simulink model "Controller_PP"  (R2021a)
settings: Solver=FixedStepDiscrete  StartTime=0.0  StopTime=inf  FixedStep=0.05  RelTol=1e-3
PostLoadFcn:
  | , if any(exist('dsrtsu_mdlpostloadfcn', 'file') == [2, 3, 6]), try dsrtsu_mdlpostloadfcn('Execute', bdroot); catch fprintf('Error in PostLoadFcn (dsrtsu_mdlpostloadfcn) for model "%s":\n %s\n', bdroot, lasterr); end, end,
model workspace (MAT data in the model file):
  DLC_kr = [-5.84862481044e-05 -6.43095507895e-05 -7.01328534794e-05 -7.5956156174e-05 -8.17794588731e-05 -8.76027615758e-05 -9.34260642811e-05 -9.92493669872e-05 -0.000105072669692 -0.000110895972393 -0.000116719275087 -0.000122542545808 ... (2080 elements, 1x2080)]
  DLC_thetar = [1.57172954906 1.57172588114 1.57172186534 1.57171750165 1.57171279008 1.57170773062 1.57170232328 1.57169656806 1.57169046495 1.57168401395 1.57167721507 1.57167006831 ... (2080 elements, 1x2080)]
  DLC_xr = [-0.00056695162723 -0.000622594591628 -0.000678008043004 -0.000733171198692 -0.000788063276025 -0.000842663492338 -0.000896951064963 -0.000950905211235 -0.00100450514849 -0.00105773009405 -0.00111055926527 -0.00116297187948 ... (2080 elements, 1x2080)]
  DLC_yr = [0.59999973213 0.659739817002 0.719479902091 0.779219987412 0.838960072984 0.898700158824 0.958440244948 1.01818033138 1.07792041812 1.1376605052 1.19740059264 1.25714068045 ... (2080 elements, 1x2080)]
  Fliter_ = 0.5
  Fliter_k = 1
  Iz = 1650
  SL_ROS_VariableLengthArrays_MaxSizes : object (value not decoded)
  a = 1
  b = 1.8
  cf = -120000
  cr = -120000
  factor_str = 0.15
  k1 = [0.258198889801 0.258198889749 0.258198889743 0.258198889805 0.258198889772 0.258198889764 0.258198889767 0.258198889768 0.258198889748 0.258198889747 0.258198889747 0.258198889747 ... (1000 elements, 1x1000)]
  k2 = [0.000225641086743 0.000451280556994 0.000676916794375 0.000902548182649 0.00112817310577 0.00135378994806 0.00157939709421 0.00180499292937 0.00203057583924 0.00225614421016 0.00248169642913 0.00270723088396 ... (1000 elements, 1x1000)]
  k3 = [1.8072435186 1.8072437178 1.80724404966 1.8072445143 1.80724511184 1.80724584231 1.80724670582 1.80724770248 1.80724883243 1.8072500958 1.80725149277 1.80725302351 ... (1000 elements, 1x1000)]
  k4 = [0.000229144738699 0.000458288056581 0.000687428532897 0.000916564747031 0.00114569527856 0.00137481870732 0.00160393361347 0.00183303857755 0.00206213218056 0.00229121300401 0.00252027963002 0.00274933064131 ... (1000 elements, 1x1000)]
  kr = [3.43040952456 5.20354947673 6.57526776383 5.89663744443 5.05963864905 4.19207203133 3.37422700169 2.64183787985 2.00068698258 1.44046440991 0.943931458435 0.491794250204 ... (89883 elements, 89883x1)]
  m = 1500
  straight_kr = [0 0 0 0 0 0 0 0 0 0 0 0 ... (10000 elements, 10000x1)]
  straight_thetar = [1.5708 1.5708 1.5708 1.5708 1.5708 1.5708 1.5708 1.5708 1.5708 1.5708 1.5708 1.5708 ... (10000 elements, 10000x1)]
  straight_xr = [0 0 0 0 0 0 0 0 0 0 0 0 ... (10000 elements, 10000x1)]
  straight_yr = [0.01 0.02 0.03 0.04 0.05 0.06 0.07 0.08 0.09 0.1 0.11 0.12 ... (10000 elements, 10000x1)]
  thetar = [0.0108871889919 0.137918447215 0.259619297152 0.371627288769 0.47112102891 0.556859678388 0.628810120477 0.687658443901 0.734398145371 0.77005371967 0.795522448239 0.811495552059 ... (89883 elements, 89883x1)]
  xr = [399944.786619 399944.805491 399944.823621 399944.841077 399944.857922 399944.874223 399944.890046 399944.905456 399944.920519 399944.935301 399944.949866 399944.964282 ... (89883 elements, 89883x1)]
  xr_init = 3407363.99438
  yr = [3406937.32043 3406937.32184 3406937.3255 3406937.33122 3406937.33879 3406937.34802 3406937.35871 3406937.37066 3406937.38366 3406937.39752 3406937.41203 3406937.427 ... (89883 elements, 89883x1)]
  yr_init = 400335.964759
undefined symbols (not defined in the file): Data, Data_SL_Info
libraries: robotlib x6, simulink_extras x3, simulink x1
(part 2 of 2)

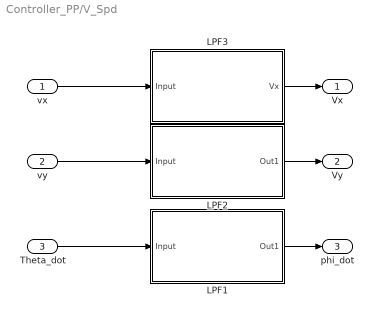
== system Controller_PP/V_Spd ==
  vx : Inport
  vy : Inport  Port=2
  Theta_dot : Inport  Port=3
  LPF1 : Subsystem  TreatAsAtomicUnit=on
  LPF2 : Subsystem  TreatAsAtomicUnit=on
  LPF3 : Subsystem  TreatAsAtomicUnit=on
  Vx : Outport  VectorParamsAs1DForOutWhenUnconnected=off
  Vy : Outport  Port=2  VectorParamsAs1DForOutWhenUnconnected=off
  phi_dot : Outport  Port=3  VectorParamsAs1DForOutWhenUnconnected=off
  wires:
  Theta_dot/1 -> LPF1/1(Input)
  LPF1/1(Out1) -> phi_dot/1
  LPF2/1(Out1) -> Vy/1
  LPF3/1(Vx) -> Vx/1
  vx/1 -> LPF3/1(Input)
  vy/1 -> LPF2/1(Input)

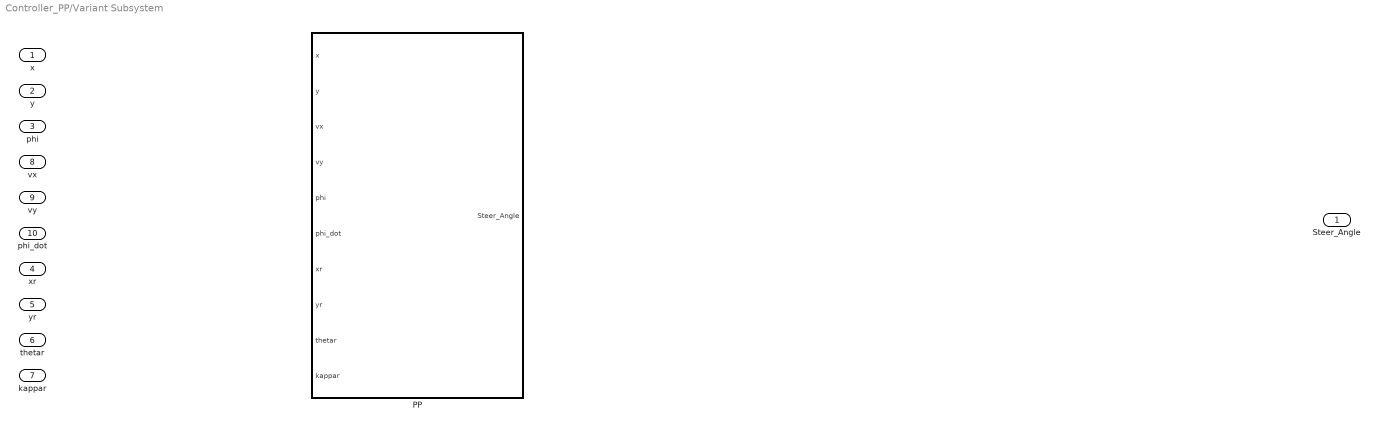
== system Controller_PP/Variant Subsystem ==
  x : Inport
  y : Inport  Port=2
  phi : Inport  Port=3
  xr : Inport  Port=4
  yr : Inport  Port=5
  thetar : Inport  Port=6
  kappar : Inport  Port=7
  vx : Inport  Port=8
  vy : Inport  Port=9
  phi_dot : Inport  Port=10
  PP : Subsystem  VariantControl=Controller == 5
  Steer_Angle : Outport  VectorParamsAs1DForOutWhenUnconnected=off

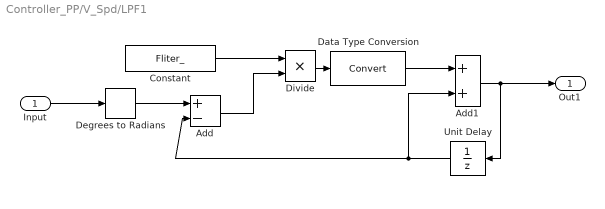
== system Controller_PP/V_Spd/LPF1 ==
  Input : Inport
  Add : Sum  Inputs=+-
  Add1 : Sum
  Constant : Constant  Value=Fliter_
  Data Type Conversion : DataTypeConversion
  Degrees to Radians : simulink_extras/Transformations/Degrees to Radians
  Divide : Product  Inputs=**
  Unit Delay : UnitDelay  SampleTime=-1  HasFrameUpgradeWarning=on
  Out1 : Outport  VectorParamsAs1DForOutWhenUnconnected=off
  wires:
  Divide/1 -> Data Type Conversion/1
  Input/1 -> Degrees to Radians/1
  Constant/1 -> Divide/1
  Add/1 -> Divide/2
  Data Type Conversion/1 -> Add1/1
  Add1/1 -> Unit Delay/1, Out1/1
  Unit Delay/1 -> Add/2, Add1/2
  Degrees to Radians/1 -> Add/1

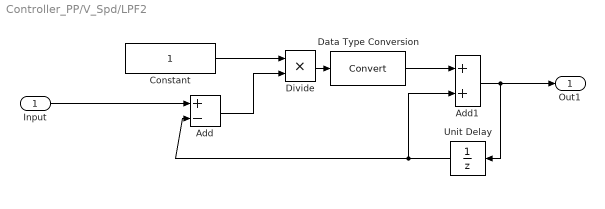
== system Controller_PP/V_Spd/LPF2 ==
  Input : Inport
  Add : Sum  Inputs=+-
  Add1 : Sum
  Constant : Constant
  Data Type Conversion : DataTypeConversion
  Divide : Product  Inputs=**
  Unit Delay : UnitDelay  SampleTime=-1  HasFrameUpgradeWarning=on
  Out1 : Outport  VectorParamsAs1DForOutWhenUnconnected=off
  wires:
  Divide/1 -> Data Type Conversion/1
  Constant/1 -> Divide/1
  Add/1 -> Divide/2
  Data Type Conversion/1 -> Add1/1
  Add1/1 -> Unit Delay/1, Out1/1
  Unit Delay/1 -> Add/2, Add1/2
  Input/1 -> Add/1

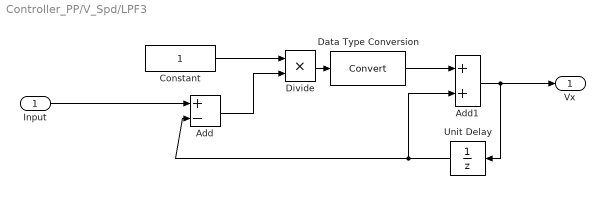
== system Controller_PP/V_Spd/LPF3 ==
  Input : Inport
  Add : Sum  Inputs=+-
  Add1 : Sum
  Constant : Constant
  Data Type Conversion : DataTypeConversion
  Divide : Product  Inputs=**
  Unit Delay : UnitDelay  SampleTime=-1  HasFrameUpgradeWarning=on
  Vx : Outport  VectorParamsAs1DForOutWhenUnconnected=off
  wires:
  Input/1 -> Add/1
  Unit Delay/1 -> Add1/2, Add/2
  Add1/1 -> Vx/1, Unit Delay/1
  Data Type Conversion/1 -> Add1/1
  Add/1 -> Divide/2
  Constant/1 -> Divide/1
  Divide/1 -> Data Type Conversion/1

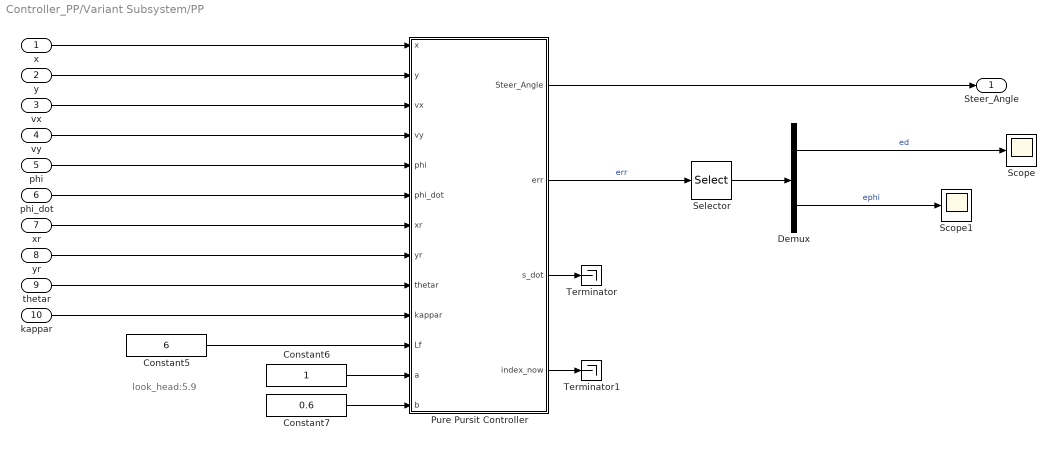
== system Controller_PP/Variant Subsystem/PP ==
  note: look_head:5.9
  x : Inport
  y : Inport  Port=2
  vx : Inport  Port=3
  vy : Inport  Port=4
  phi : Inport  Port=5
  phi_dot : Inport  Port=6
  xr : Inport  Port=7
  yr : Inport  Port=8
  thetar : Inport  Port=9
  kappar : Inport  Port=10
  Constant5 : Constant  Value=6
  Constant6 : Constant
  Constant7 : Constant  Value=0.6
  Demux : Demux  Outputs=2
  Pure Pursit Controller : MATLAB Function  TreatAsAtomicUnit=on
  Scope : Scope
  Scope1 : Scope
  Selector : Selector  InputPortWidth=4  IndexOptions=Index vector (dialog)  Indices=[1 3]  OutputSizes=1
  Terminator : Terminator
  Terminator1 : Terminator
  Steer_Angle : Outport
  wires:
  phi_dot/1 -> Pure Pursit Controller/6(phi_dot)
  Pure Pursit Controller/3(s_dot) -> Terminator/1
  Selector/1 -> Demux/1
  Constant7/1 -> Pure Pursit Controller/13(b)
  Constant5/1 -> Pure Pursit Controller/11(Lf)
  Demux/2 -> Scope1/1  "ephi"
  vx/1 -> Pure Pursit Controller/3(vx)
  y/1 -> Pure Pursit Controller/2(y)
  thetar/1 -> Pure Pursit Controller/9(thetar)
  xr/1 -> Pure Pursit Controller/7(xr)
  Constant6/1 -> Pure Pursit Controller/12(a)
  vy/1 -> Pure Pursit Controller/4(vy)
  yr/1 -> Pure Pursit Controller/8(yr)
  Pure Pursit Controller/2(err) -> Selector/1  "err"
  Demux/1 -> Scope/1  "ed"
  x/1 -> Pure Pursit Controller/1(x)
  kappar/1 -> Pure Pursit Controller/10(kappar)
  Pure Pursit Controller/1(Steer_Angle) -> Steer_Angle/1
  phi/1 -> Pure Pursit Controller/5(phi)
  Pure Pursit Controller/4(index_now) -> Terminator1/1

== matlab function Controller_PP/MATLAB Function1 ==
  data: u input; y output; acc input; speed input
function y = fcn(u,acc, speed)
if u == 1
    y = 0;
elseif u == 2
    y = acc; 
else
    y = speed;
end

== matlab function Controller_PP/MATLAB Function ==
  data: Traj input; xr output; yr output; thetar output; kappar output
function [xr,yr,thetar,kappar] = fcn(Traj)
xr = zeros(1,501);
yr = zeros(1,501);
thetar = zeros(1,501);
kappar = zeros(1,501);

xr(:) = Traj(1:501);
yr(:) = Traj(502:1002);
thetar(:) = Traj(1003:1503);
kappar(:) = Traj(1504:2004);
end

== matlab function Controller_PP/MATLAB Function2 ==
  data: u input; y output; left_factor input; right_factor input
function y = fcn(u,left_factor,right_factor)
if u>=110 && u<=130
    y = u;
elseif u>=130 && u<=240
    y = left_factor*u;
else
    y = right_factor*u;
    
end
end

== stateflow chart Controller_PP/Chart ==
  state ACC
    en:
    OutPut = 2;
  state wait
  state Init
    en:
    OutPut = InPut;
  state Stop
    en:
    OutPut = 1;
  (default) -> Init
  wait -> ACC : after(10,sec)
  Init -> wait [order 1] : [InPut == 2]
  ACC -> Stop : [InPut == 1&& after(2,sec)]
  Init -> (junction 7) [order 2] : [InPut == 1&&after(2,sec)]
  (junction 7) -> Stop
  data: InPut input; OutPut output

== matlab function Controller_PP/Variant Subsystem/PP/Pure Pursit Controller ==
  settings: updateMethod=DISCRETE
  data: x input; Steer_Angle output; y input; vx input; vy input; phi input; phi_dot input; xr input; yr input; thetar input; kappar input; err output; s_dot output; index_now output; Lf input; a input; b input
function [Steer_Angle,err,s_dot,index_now] = fcn(x,y,vx,vy,phi,phi_dot,xr,yr,thetar,kappar, Lf,a,b)
n=length(xr);
dmin=1;
d_min_last = 1;
for i = 1:n
    d_min = (x-xr(i))^2+(y-yr(i))^2;
    if d_min < d_min_last
        dmin = i;
        d_min_last = d_min;
    end
end
    tor=[cos(thetar(dmin));sin(thetar(dmin))];
    nor=[-sin(thetar(dmin));cos(thetar(dmin))];
    d_err=[x-xr(dmin);y-yr(dmin)];
    ed=nor'*d_err;
    es=tor'*d_err;
    projection_point_thetar=thetar(dmin)+kappar(dmin)*es;
    ed_dot=vy*cos(phi-projection_point_thetar)+vx*sin(phi-projection_point_thetar);
    ephi=sin(phi-projection_point_thetar);
    s_dot1=vx*cos(phi-projection_point_thetar)-vy*sin(phi-projection_point_thetar);
    s_dot=s_dot1/(1-kappar(dmin)*ed);
    ephi_dot=phi_dot-kappar(dmin)*s_dot;
    kr=kappar(dmin);
    err=[ed;ed_dot;ephi;ephi_dot]; 
    
    L = 0.0; %Look ahead distance
    index_now = dmin;
    while Lf > L && (index_now + 1) < n                %计算思想：找到与当前位置最近的那个全局路径参考点前方预设预瞄距离的点，返回其在全局路径上的矩阵索引位。确定预瞄点
        L=sqrt((x-xr(index_now))^2+(y-yr(index_now))^2);
       % L = norm(curpos(1,1:2)-repos(index,1:2));
        index_now =index_now+1;
        %disp("%d",ind)
    end

    xr_LD =xr(index_now);%确定要跟踪的预瞄点坐标
    yr_LD =yr(index_now);
    Lateral_Err = (a+b)*sin(atan2((yr_LD-y),(xr_LD-x))  - phi);
    Steer_Angle = atan(2*Lateral_Err/Lf);
 
end
